simulink model "QR_select"  (R2024a)
settings: Solver=VariableStepAuto  StartTime=0.0  StopTime=10.0  RelTol=1e-3
values from neighbouring files (symbols this model uses):
  A = double(subs(A_sym, param, param_num))    [AB_solve.m]
  B = double(subs(B_sym, param, param_num))    [AB_solve.m]
  C = eye(10)    [QR_select_var.m]
  D = zeros(10, 4)    [QR_select_var.m]
  K = lqr(A, B, Q, R)    [QR_select_var.m]
  x_init = [1; 0; 0; 0; 0; 0; 0; 0; 0; 0]    [QR_select_var.m]
  x_set = [0; 0; 0; 0; 0; 0; 0; 0; 0; 0]    [QR_select_var.m]
settings Model: Creator=dokee  LastModifiedBy=dokee

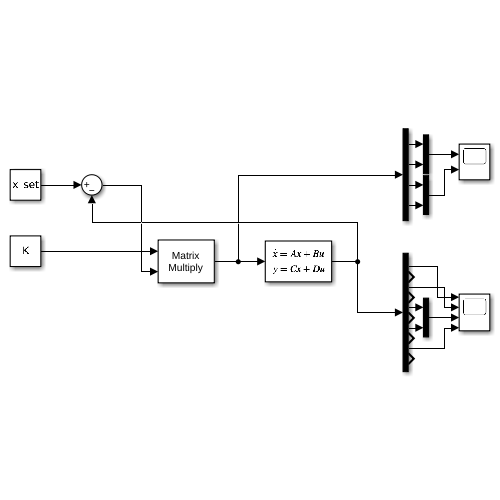
[thumbnail: Simulink's stored preview of the top-level diagram]
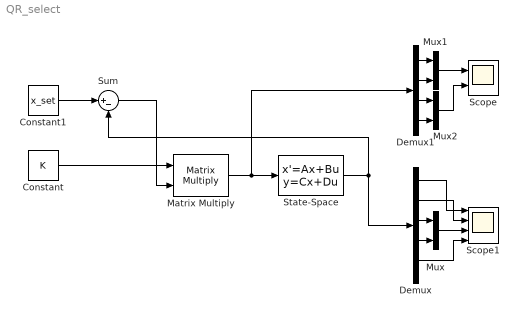
== system QR_select ==
  Constant : Constant  Value=K
  Constant1 : Constant  Value=x_set
  Demux : Demux  Outputs=10
  Demux1 : Demux
  Matrix Multiply : Product  Multiplication=Matrix(*)
  Mux : Mux  Inputs=2
  Mux1 : Mux  Inputs=2
  Mux2 : Mux  Inputs=2
  Scope : Scope  NumInputPorts=2
  Scope1 : Scope  NumInputPorts=4
  State-Space : StateSpace  A=A  B=B  C=C  D=D  InitialCondition=x_init
  Sum : Sum  Inputs=|+-
  wires:
  Constant/1 -> Matrix Multiply/1
  Matrix Multiply/1 -> Demux1/1, State-Space/1
  State-Space/1 -> Demux/1, Sum/2
  Constant1/1 -> Sum/1
  Sum/1 -> Matrix Multiply/2
  Demux/1 -> Scope1/1
  Demux/3 -> Scope1/2
  Demux/5 -> Mux/1
  Demux/7 -> Mux/2
  Mux/1 -> Scope1/3
  Demux/9 -> Scope1/4
  Demux1/1 -> Mux1/1
  Demux1/2 -> Mux1/2
  Demux1/3 -> Mux2/1
  Demux1/4 -> Mux2/2
  Mux1/1 -> Scope/1
  Mux2/1 -> Scope/2
